simulink model "questC_custom_model"  (R2018a)
settings: Solver=VariableStepAuto  StartTime=0.0  StopTime=5  RelTol=1e-3
values from neighbouring files (symbols this model uses):
  A = [0 1 0 0; 20.6 0 0 0; 0 0 0 1; -.5 0 0 0]    [InvertedPendulum.m]
  B = [0; -1; 0; .5]    [InvertedPendulum.m]
  C = [1 0 0 0; 0 0 1 0]    [InvertedPendulum.m]
  K = place(A, B, p)    [InvertedPendulum.m]
  x0 = [-.2; -.06; .01; .3]    [InvertedPendulum.m]
settings Model: Creator=patsa  LastModifiedBy=patsa

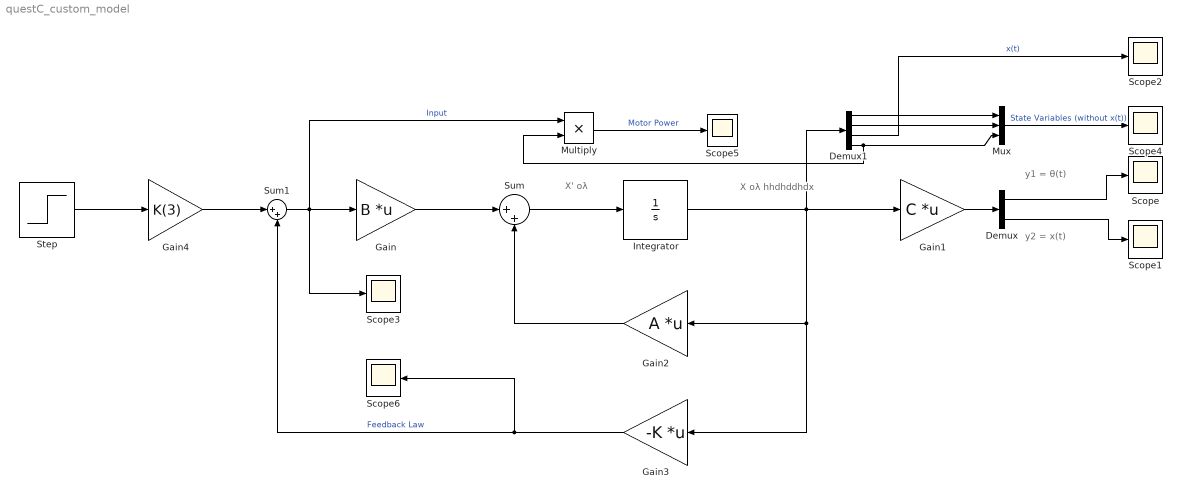
== system questC_custom_model ==
  note: X' ολ
  note: X ολ
      |
      | hhdhddhdx
  note: y2 = x(t)
  note: y1 = θ(t)
  Demux : Demux  Outputs=2
  Demux1 : Demux
  Gain : Gain  Gain=B  Multiplication=Matrix(K*u)
  Gain1 : Gain  Gain=C  Multiplication=Matrix(K*u)
  Gain2 : Gain  Gain=A  Multiplication=Matrix(K*u)
  Gain3 : Gain  Gain=-K  Multiplication=Matrix(K*u)
  Gain4 : Gain  Gain=K(3)
  Integrator : Integrator  InitialCondition=x0
  Multiply : Product
  Mux : Mux  Inputs=3
  Scope{,1..6} (7 alike) : Scope
  Step : Step  Time=0  SampleTime=0
  Sum : Sum  Inputs=|++
  Sum1 : Sum  Inputs=|++
  wires:
  Demux/2 -> Scope1/1
  Integrator/1 -> Gain3/1, Gain2/1, Demux1/1, Gain1/1
  Gain2/1 -> Sum/2
  Gain3/1 -> Sum1/2, Scope6/1  "Feedback Law"
  Gain1/1 -> Demux/1
  Demux/1 -> Scope/1
  Gain/1 -> Sum/1
  Sum/1 -> Integrator/1
  Step/1 -> Gain4/1
  Gain4/1 -> Sum1/1
  Sum1/1 -> Multiply/1, Scope3/1, Gain/1  "Input"
  Demux1/1 -> Mux/1
  Demux1/2 -> Mux/2
  Demux1/4 -> Multiply/2, Mux/3
  Mux/1 -> Scope4/1  "State Variables (without x(t))"
  Demux1/3 -> Scope2/1  "x(t)"
  Multiply/1 -> Scope5/1  "Motor Power"
